simulink model "labcartcola"  (Simulink 6.1)
settings: Solver=ode1  SolverMode=SingleTasking  StartTime=0.0  StopTime=inf  FixedStep=0.001  RelTol=1e-3
libraries: qctools x3
settings Model: LastModifiedBy=localadmin  ExtModeArmWhenConnect=off  BufferReuse=off
settings ConfigSet: SimulationMode=external
settings OptimizationCC: BooleanDataType=off  OptimizeBlockIOStorage=off  BufferReuse=off  ExpressionFolding=off  LocalBlockOutputs=off
settings DebuggingCC: SolverPrmCheckMsg=warning
settings RTWCC: SystemTargetFile=wincon.tlc  MakeCommand=make_wc  TemplateMakefile=wc_default_tmf  Description=WinCon Target  ProcessScript=wincon_make_rtw_hook
settings STFCustomTargetCC: TargetFcnLib=ansi_tfl_tmw.mat  GenFloatMathFcnCalls=ANSI_C  ModelReferenceCompliant=off  SystemTargetFile=wincon.tlc
settings GRTTargetCC: ModelReferenceCompliant=off  MatFileLogging=off  ExtMode=on  ExtModeTransport=2  ExtModeMexFile=wc_comm
settings CustomProperty: Value=on

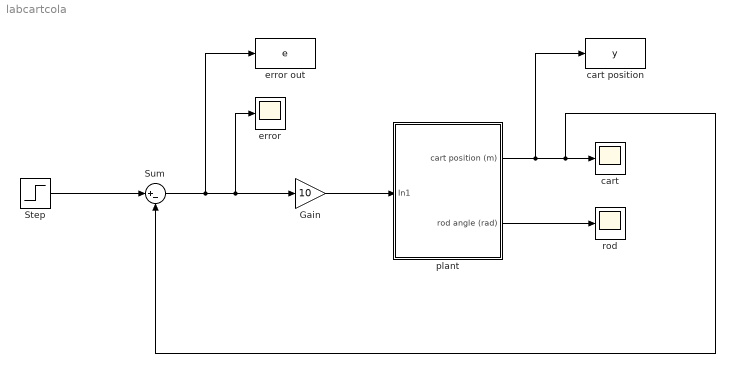
== system labcartcola ==
  Gain : Gain  Gain=10
  Step : Step  Time=0  After=0.4  SampleTime=0
  Sum : Sum  Inputs=|+-
  cart : Scope
  cart position : ToWorkspace  VariableName=y  SampleTime=-1  SaveFormat=Structure
  error : Scope
      settings: SaveName=ScopeData3
  error out : ToWorkspace  VariableName=e  SampleTime=-1  SaveFormat=Structure
  plant : Subsystem
  rod : Scope
  wires:
  plant/2(rod angle (rad)) -> rod/1
  plant/1(cart position (m)) -> Sum/2, cart/1, cart position/1
  Sum/1 -> error/1, Gain/1, error out/1
  Gain/1 -> plant/1(In1)
  Step/1 -> Sum/1

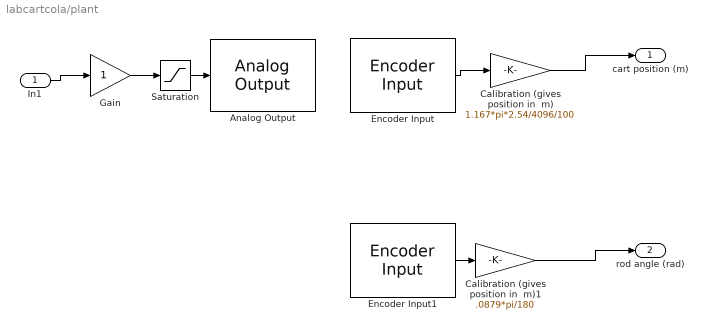
== system labcartcola/plant ==
  In1 : Inport  Port=1  LatchInput=off
  Analog Output : qctools/Quanser Q4 Series/Analog Output  boardNumber=0  channels=0  modesVect=0  rangesVect=10  initialVect=0  finalVect=0  sampleTime=-1  inputVolts=on  simulationOutput=off
  Calibration (gives position in  m) : Gain  Gain=1.167*pi*2.54/4096/100  SaturateOnIntegerOverflow=on
  Calibration (gives position in  m)1 : Gain  Gain=.0879*pi/180  SaturateOnIntegerOverflow=on
  Encoder Input : qctools/Quanser Q4 Series/Encoder Input  boardNumber=0  channels=0  initial=0  preserveCounts=off  sampleTime=default_sample_time  quadratureStr=4X  modeStr=Normal  flagString=FLG1 is IDX and FLG2 is E  prescale=1  frequency=16666666.6667  use33MHzClock=off  bcd=off  enableIndex=on  synchronousIndex=on  indexPolarity=on  reloadOnIndex=off  simulationInput=off
  Encoder Input1 : qctools/Quanser Q4 Series/Encoder Input  boardNumber=0  channels=1  initial=0  preserveCounts=off  sampleTime=default_sample_time  quadratureStr=4X  modeStr=Normal  flagString=FLG1 is IDX and FLG2 is E  prescale=1  frequency=16666666.6667  use33MHzClock=off  bcd=off  enableIndex=on  synchronousIndex=on  indexPolarity=on  reloadOnIndex=off  simulationInput=off
  Gain : Gain  SaturateOnIntegerOverflow=on
  Saturation : Saturate  UpperLimit=6  LowerLimit=-6
  cart position (m) : Outport
  rod angle (rad) : Outport  Port=2
  wires:
  Encoder Input/1 -> Calibration (gives position in  m)/1
  Calibration (gives position in  m)/1 -> cart position (m)/1
  Calibration (gives position in  m)1/1 -> rod angle (rad)/1
  Encoder Input1/1 -> Calibration (gives position in  m)1/1
  Saturation/1 -> Analog Output/1
  In1/1 -> Gain/1
  Gain/1 -> Saturation/1
